simulink model "CC to ACC Final"  (R2024b)
settings: Solver=VariableStepAuto  StartTime=0.0  StopTime=40  RelTol=1e-3
undefined symbols (not defined in the file or in its folder): Sim3dSensor
libraries: drivingscenarioandsensors x5, sim3dautolib x2, sim3dcameralib x1, sim3dlib x1
(part 1 of 4)
settings Model: Creator=Harshal  LastModifiedBy=PARSYSTEM

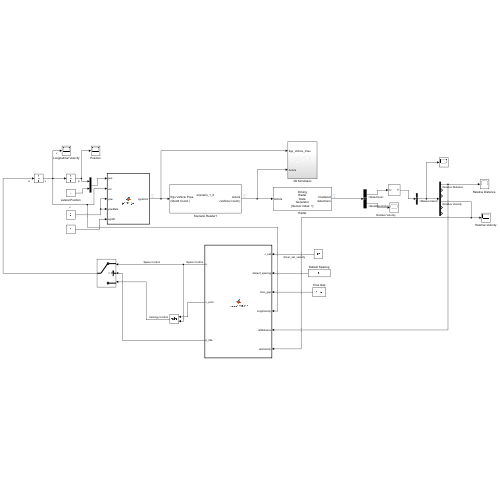
[thumbnail: Simulink's stored preview of the top-level diagram]
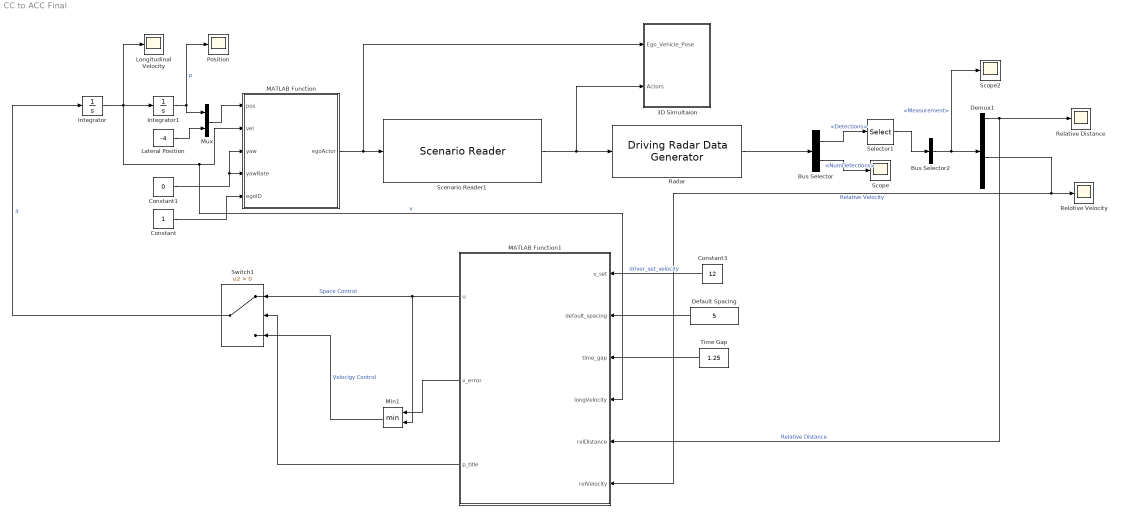
== system CC to ACC Final ==
  3D Simultaion : Subsystem
  Bus Selector : BusSelector  OutputSignals=Detections,NumDetections
  Bus Selector2 : BusSelector  OutputSignals=Measurement
  Constant : Constant
  Constant1 : Constant  Value=0
  Constant3 : Constant  Value=12
  Default Spacing : Constant  Value=5  SampleTime=0
  Demux1 : Demux  Outputs=6
  Integrator : Integrator
  Integrator1 : Integrator
  Lateral Position : Constant  Value=-4
  Longitudinal Velocity : Scope
  MATLAB Function : MATLAB Function  TreatAsAtomicUnit=on
  MATLAB Function1 : MATLAB Function  TreatAsAtomicUnit=on
  Min1 : MinMax  Inputs=2
  Mux : Mux  Inputs=2
  Position : Scope
